simulink model "gps2"  (Simulink 7.5)
settings: Solver=ode45  StartTime=0.0  StopTime=10.0  RelTol=1e-3
libraries: dspsrcs4 x1
settings Model: Creator=sisa  LastModifiedBy=sisa

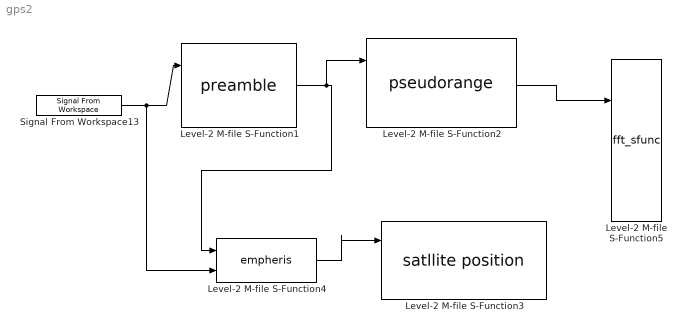
== system gps2 ==
  Level-2 M-file S-Function1 : M-S-Function  FunctionName=preamble
  Level-2 M-file S-Function2 : M-S-Function  FunctionName=pseudorange
  Level-2 M-file S-Function3 : M-S-Function  FunctionName=satllite position
  Level-2 M-file S-Function4 : M-S-Function  FunctionName=empheris
  Level-2 M-file S-Function5 : M-S-Function  FunctionName=fft_sfunc
  Signal From Workspace13 : dspsrcs4/Signal From Workspace  SystemSampleTime=-1  X=trackingresults  Ts=1  nsamps=1  OutputAfterFinalValue=Setting to zero  ignoreOrWarnInputAndFrameLengths=off
  wires:
  Signal From Workspace13/1 -> Level-2 M-file S-Function1/1, Level-2 M-file S-Function4/2
  Level-2 M-file S-Function1/1 -> Level-2 M-file S-Function2/1, Level-2 M-file S-Function4/1
  Level-2 M-file S-Function4/1 -> Level-2 M-file S-Function3/1
  Level-2 M-file S-Function2/1 -> Level-2 M-file S-Function5/1
